simulink model "DOA_rearanged_2020a"  (R2020a)
settings: Solver=ode4  StartTime=0.0  StopTime=0.25  RelTol=1e-3
values from neighbouring files (symbols this model uses):
  f_range = [20e3 45e3]    [Init.m]
  FFT_LENGTH = 256    [Init.m]
  Sampling_rate = 256e3    (= 256000)    [Init.m]
undefined symbols (not defined in the file or in its folder): Coeff_han
libraries: dspsigops x25, dsphdlmathfun x4, dsphdlxfrm x4, simulink x1, hdlsllib x1
settings Model: Creator=tigro  LastModifiedBy=franc
settings OptimizationCC: BlockReduction=off  ConditionallyExecuteInputs=off  DefaultParameterBehavior=Inlined
settings DebuggingCC: AlgebraicLoopMsg=error  ParameterOverflowMsg=none  AllowAutomaticUnitConversions=off
settings HardwareCC: ProdBitPerPointer=32  ProdBitPerSizeT=32  ProdBitPerPtrDiffT=32  ProdLargestAtomicFloat=None  ProdIntDivRoundTo=Undefined  ProdEndianess=Unspecified  ProdWordSize=32  ProdHWDeviceType=ASIC/FPGA->ASIC/FPGA  TargetBitPerPointer=64  TargetBitPerSizeT=64  TargetBitPerPtrDiffT=64  TargetLongLongMode=on  TargetIntDivRoundTo=Zero  TargetEndianess=LittleEndian  TargetWordSize=64  TargetHWDeviceType=Custom Processor->MATLAB Host Computer  ProdEqTarget=off

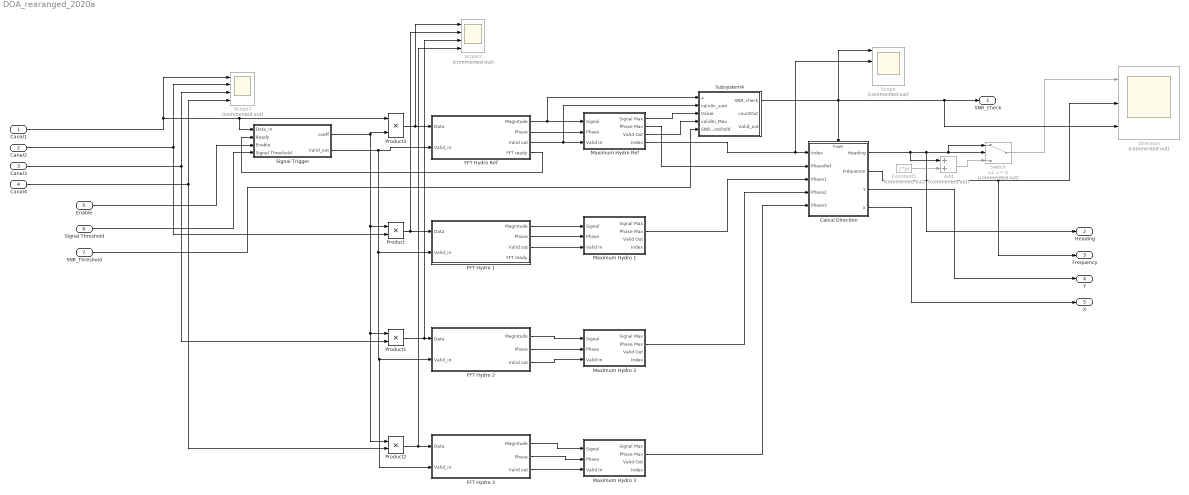
== system DOA_rearanged_2020a ==
  Canal1 : Inport  OutDataTypeStr=uint16
  Canal2 : Inport  Port=2  OutDataTypeStr=uint16
  Canal3 : Inport  Port=3  OutDataTypeStr=uint16
  Canal4 : Inport  Port=4  OutDataTypeStr=uint16
  Enable : Inport  Port=5  SampleTime=1/Sampling_rate
  Signal Threshold : Inport  Port=6
  SNR_Threshold : Inport  Port=7  OutDataTypeStr=uint16
  Add : Sum  Commented=on
  Calcul Direction : Subsystem
  Constant5 : Constant  Commented=on  Value=2*pi
  Direction : Scope  Commented=on  NumInputPorts=3
  FFT Hydro 1 : Subsystem
  FFT Hydro 2 : Subsystem
  FFT Hydro 3 : Subsystem
  FFT Hydro Ref : Subsystem
  Maximum Hydro 1 : Subsystem
  Maximum Hydro 2 : Subsystem
  Maximum Hydro 3 : Subsystem
  Maximum Hydro Ref : Subsystem
  Product{,1..3} (4 alike) : Product
  Scope : Scope  Commented=on  NumInputPorts=4
  Scope1 : Scope  Commented=on  NumInputPorts=4
  Scope2 : Scope  Commented=on  NumInputPorts=4
  Signal Trigger : Subsystem  TreatAsAtomicUnit=on
  Subsystem4 : Subsystem
  Switch : Switch  Commented=on
  SNR_Check : Outport
  Heading : Outport  Port=2
  Frequency : Outport  Port=3
  Y : Outport  Port=4
  X : Outport  Port=5
  wires:
  Maximum Hydro Ref/1(Signal Max) -> Subsystem4/3(" Value")
  Maximum Hydro Ref/4(Index) -> Scope/2, Calcul Direction/1(Index)
  Calcul Direction/1(Heading) -> Heading/1, Switch/2, Switch/1, Add/1
  Add/1 -> Switch/3
  Constant5/1 -> Add/2
  Product3/1 -> Scope2/1, FFT Hydro Ref/1(Data)
  Product/1 -> Scope2/2, FFT Hydro 1/1(Data)
  Product1/1 -> Scope2/3, FFT Hydro 2/1(Data)
  Product2/1 -> Scope2/4, FFT Hydro 3/1(Data)
  FFT Hydro Ref/2(Phase) -> Maximum Hydro Ref/2(Phase)
  Maximum Hydro Ref/2(Phase Max) -> Calcul Direction/2(PhaseRef)
  Maximum Hydro 1/2(Phase Max) -> Calcul Direction/3(Phase1)
  Maximum Hydro 2/2(Phase Max) -> Calcul Direction/4(Phase2)
  Maximum Hydro 3/2(Phase Max) -> Calcul Direction/5(Phase3)
  Signal Trigger/1(coeff) -> Product3/2, Product/1, Product1/1, Product2/1
  FFT Hydro 1/1(Magnitude) -> Maximum Hydro 1/1(Signal)
  FFT Hydro 1/2(Phase) -> Maximum Hydro 1/2(Phase)
  FFT Hydro 1/3(Valid out) -> Maximum Hydro 1/3(Valid In)
  FFT Hydro 2/2(Phase) -> Maximum Hydro 2/2(Phase)
  Maximum Hydro Ref/3(Valid Out) -> Subsystem4/4(validIn_Max)
  FFT Hydro Ref/4(FFT ready) -> Signal Trigger/2(Ready)
  FFT Hydro Ref/3(Valid out) -> Maximum Hydro Ref/3(Valid In), Subsystem4/2(validIn_sum)
  Calcul Direction/2(Fréquence) -> Frequency/1, Direction/2
  Calcul Direction/3(Y) -> Y/1
  Calcul Direction/4(X) -> X/1
  Switch/1 -> Direction/1
  FFT Hydro Ref/1(Magnitude) -> Subsystem4/1(a), Maximum Hydro Ref/1(Signal)
  Subsystem4/1(SNR_check) -> SNR_Check/1, Direction/3, Scope/1, Calcul Direction/Trigger
  Enable/1 -> Signal Trigger/3(Enable)
  Signal Threshold/1 -> Signal Trigger/4(Signal Threshold)
  SNR_Threshold/1 -> Subsystem4/5(SNR_Threshold)
  Signal Trigger/2(Valid_out) -> FFT Hydro 1/2(Valid_in), FFT Hydro 3/2(Valid_in), FFT Hydro 2/2(Valid_in), FFT Hydro Ref/2(Valid_in)
  Canal1/1 -> Scope1/1, Product3/1, Signal Trigger/1(Data_in)
  Canal2/1 -> Product/2, Scope1/2
  Canal3/1 -> Product1/2, Scope1/3
  Canal4/1 -> Product2/2, Scope1/4
  FFT Hydro 2/1(Magnitude) -> Maximum Hydro 2/1(Signal)
  FFT Hydro 2/3(Valid out) -> Maximum Hydro 2/3(Valid In)
  FFT Hydro 3/1(Magnitude) -> Maximum Hydro 3/1(Signal)
  FFT Hydro 3/2(Phase) -> Maximum Hydro 3/2(Phase)
  FFT Hydro 3/3(Valid out) -> Maximum Hydro 3/3(Valid In)

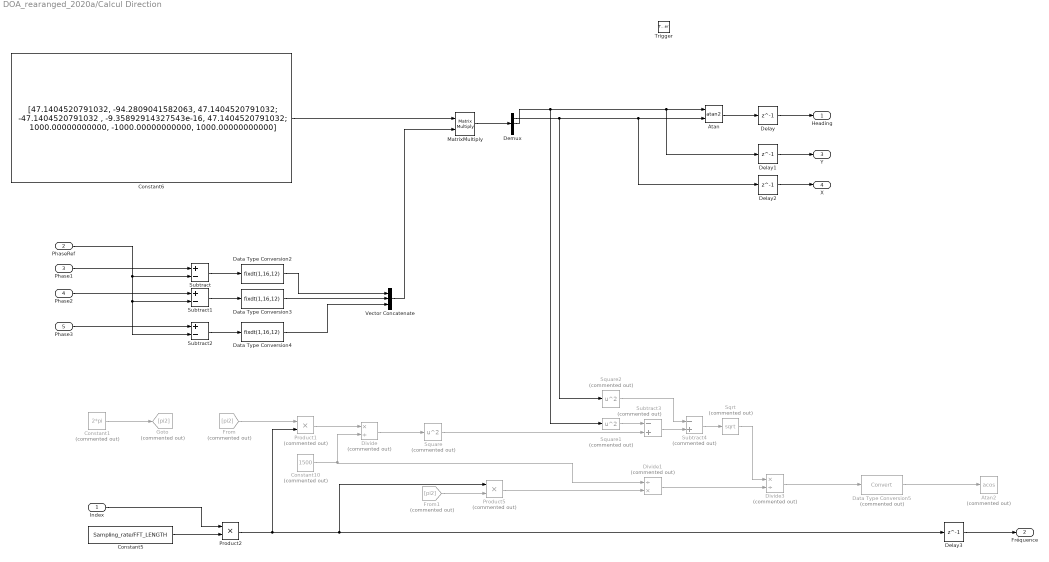
== system DOA_rearanged_2020a/Calcul Direction ==
  Index : Inport
  PhaseRef : Inport  Port=2
  Phase1 : Inport  Port=3
  Phase2 : Inport  Port=4
  Phase3 : Inport  Port=5
  Trigger : TriggerPort  VariantControl=Variant  PortDimensions=1
  Atan : Trigonometry  Operator=atan2  ApproximationMethod=CORDIC  OutputSignalType=real
  Atan2 : Trigonometry  Commented=on  Operator=acos  ApproximationMethod=CORDIC  OutputSignalType=real
  Constant1 : Constant  Commented=on  Value=2*pi  OutDataTypeStr=fixdt(0,7,3)  SampleTime=-1
  Constant10 : Constant  Commented=on  Value=1500  OutDataTypeStr=fixdt(0,11)  SampleTime=-1
  Constant5 : Constant  Value=Sampling_rate/FFT_LENGTH  OutDataTypeStr=fixdt(0,10)  SampleTime=-1
  Constant6 : Constant  Value=|  VectorParams1D=off  OutDataTypeStr=fixdt(1,15,7)  SampleTime=-1
      | [47.1404520791032,    -94.2809041582063,    47.1404520791032;
      | -47.1404520791032 ,   -9.35892914327543e-16,    47.1404520791032;
      | 1000.00000000000,   -1000.00000000000,    1000.00000000000]
  Data Type Conversion2 : DataTypeConversion  OutDataTypeStr=fixdt(1,16,12)
  Data Type Conversion3 : DataTypeConversion  OutDataTypeStr=fixdt(1,16,12)
  Data Type Conversion4 : DataTypeConversion  OutDataTypeStr=fixdt(1,16,12)
  Data Type Conversion5 : DataTypeConversion  Commented=on
  Delay{,1..3} (4 alike) : Delay  DelayLength=1
  Demux : Demux  Outputs=3
  Divide : Product  Commented=on  Inputs=*/
  Divide1 : Product  Commented=on  Inputs=/*
  Divide3 : Product  Commented=on  Inputs=*/
  From : From  Commented=on  GotoTag=pi2
  From1 : From  Commented=on  GotoTag=pi2
  Goto : Goto  Commented=on  GotoTag=pi2
  MatrixMultiply : Product  Multiplication=Matrix(*)
  Product1 : Product  Commented=on
  Product2 : Product
  Product5 : Product  Commented=on
  Sqrt : Sqrt  Commented=on  SaturateOnIntegerOverflow=on
  Square : Math  Commented=on  Operator=square  SignedPower=on  RndMeth=Zero  SaturateOnIntegerOverflow=on
  Square1 : Math  Commented=on  Operator=square  SignedPower=on  RndMeth=Zero  SaturateOnIntegerOverflow=on
  Square2 : Math  Commented=on  Operator=square  SignedPower=on  RndMeth=Zero  SaturateOnIntegerOverflow=on
  Subtract : Sum  Inputs=+-
  Subtract1 : Sum  Inputs=+-
  Subtract2 : Sum  Inputs=+-
  Subtract3 : Sum  Commented=on  Inputs=-+
  Subtract4 : Sum  Commented=on  Inputs=-+
  Vector Concatenate : Concatenate  NumInputs=3  Mode=Multidimensional array
  Heading : Outport  InitialOutput=0
  Fréquence : Outport  Port=2  InitialOutput=0
  Y : Outport  Port=3  InitialOutput=0
  X : Outport  Port=4  InitialOutput=0
  wires:
  Vector Concatenate/1 -> MatrixMultiply/2
  MatrixMultiply/1 -> Demux/1
  PhaseRef/1 -> Subtract/2, Subtract1/2, Subtract2/2
  Phase1/1 -> Subtract/1
  Phase2/1 -> Subtract1/1
  Phase3/1 -> Subtract2/1
  Subtract/1 -> Data Type Conversion2/1
  Subtract1/1 -> Data Type Conversion3/1
  Subtract2/1 -> Data Type Conversion4/1
  Constant6/1 -> MatrixMultiply/1
  Sqrt/1 -> Divide3/1
  Divide/1 -> Square/1
  From/1 -> Product1/1
  Demux/2 -> Square1/1, Delay1/1, Atan/1
  Constant1/1 -> Goto/1
  Divide1/1 -> Divide3/2
  Product5/1 -> Divide1/2
  From1/1 -> Product5/2
  Constant10/1 -> Divide/2, Divide1/1
  Subtract3/1 -> Subtract4/2
  Product1/1 -> Divide/1
  Square1/1 -> Subtract3/1
  Square/1 -> Subtract3/2
  Subtract4/1 -> Sqrt/1
  Constant5/1 -> Product2/2
  Index/1 -> Product2/1
  Square2/1 -> Subtract4/1
  Demux/1 -> Square2/1, Delay2/1, Atan/2
  Divide3/1 -> Data Type Conversion5/1
  Product2/1 -> Delay3/1, Product5/1, Product1/2
  Data Type Conversion2/1 -> Vector Concatenate/1
  Data Type Conversion3/1 -> Vector Concatenate/2
  Data Type Conversion4/1 -> Vector Concatenate/3
  Data Type Conversion5/1 -> Atan2/1
  Atan/1 -> Delay/1
  Delay/1 -> Heading/1
  Delay2/1 -> X/1
  Delay1/1 -> Y/1
  Delay3/1 -> Fréquence/1

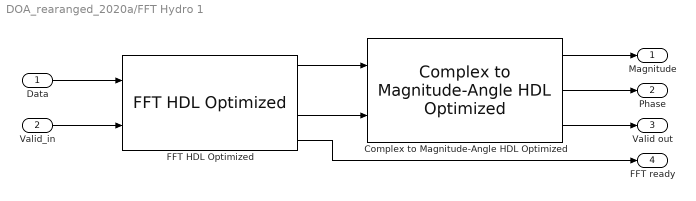
== system DOA_rearanged_2020a/FFT Hydro 1 ==
  Data : Inport
  Valid_in : Inport  Port=2
  Complex to Magnitude-Angle HDL Optimized : dsphdlmathfun/Complex to Magnitude-Angle HDL Optimized  NumIterationsSource=Property  NumIterations=CORDIC_Estimation  OutputFormat=Magnitude and angle  AngleFormat=Radians  ScaleOutput=on  SimulateUsing=Code generation
      settings: SourceProductBaseCode=DS
  FFT HDL Optimized : dsphdlxfrm/FFT HDL Optimized  FFTLength=FFT_LENGTH  Architecture=Burst Radix 2  ComplexMultiplication=Use 3 multipliers and 5 adders  BitReversedOutput=off  BitReversedInput=off  Normalize=on  SimulateUsing=Code generation  RoundingMethod=Floor  ResetInputPort=off  StartOutputPort=off  EndOutputPort=on
      settings: SourceProductBaseCode=DS
  Magnitude : Outport
  Phase : Outport  Port=2
  Valid out : Outport  Port=3
  FFT ready : Outport  Port=4
  wires:
  Valid_in/1 -> FFT HDL Optimized/2
  FFT HDL Optimized/1 -> Complex to Magnitude-Angle HDL Optimized/1
  Complex to Magnitude-Angle HDL Optimized/1 -> Magnitude/1
  Complex to Magnitude-Angle HDL Optimized/2 -> Phase/1
  Data/1 -> FFT HDL Optimized/1
  FFT HDL Optimized/3 -> Complex to Magnitude-Angle HDL Optimized/2
  Complex to Magnitude-Angle HDL Optimized/3 -> Valid out/1
  FFT HDL Optimized/4 -> FFT ready/1

== system DOA_rearanged_2020a/FFT Hydro 2 ==
  Data : Inport
  Valid_in : Inport  Port=2
  Complex to Magnitude-Angle HDL Optimized : dsphdlmathfun/Complex to Magnitude-Angle HDL Optimized  NumIterationsSource=Property  NumIterations=CORDIC_Estimation  OutputFormat=Magnitude and angle  AngleFormat=Radians  ScaleOutput=on  SimulateUsing=Code generation
      settings: SourceProductBaseCode=DS
  FFT HDL Optimized : dsphdlxfrm/FFT HDL Optimized  FFTLength=FFT_LENGTH  Architecture=Burst Radix 2  ComplexMultiplication=Use 3 multipliers and 5 adders  BitReversedOutput=off  BitReversedInput=off  Normalize=on  SimulateUsing=Code generation  RoundingMethod=Floor  ResetInputPort=off  StartOutputPort=off  EndOutputPort=off
      settings: SourceProductBaseCode=DS
  Magnitude : Outport
  Phase : Outport  Port=2
  Valid out : Outport  Port=3
  wires:
  Valid_in/1 -> FFT HDL Optimized/2
  FFT HDL Optimized/1 -> Complex to Magnitude-Angle HDL Optimized/1
  FFT HDL Optimized/2 -> Complex to Magnitude-Angle HDL Optimized/2
  Complex to Magnitude-Angle HDL Optimized/1 -> Magnitude/1
  Complex to Magnitude-Angle HDL Optimized/3 -> Valid out/1
  Complex to Magnitude-Angle HDL Optimized/2 -> Phase/1
  Data/1 -> FFT HDL Optimized/1

== system DOA_rearanged_2020a/FFT Hydro 3 ==
  Data : Inport
  Valid_in : Inport  Port=2
  Complex to Magnitude-Angle HDL Optimized : dsphdlmathfun/Complex to Magnitude-Angle HDL Optimized  NumIterationsSource=Property  NumIterations=CORDIC_Estimation  OutputFormat=Magnitude and angle  AngleFormat=Radians  ScaleOutput=on  SimulateUsing=Code generation
      settings: SourceProductBaseCode=DS
  FFT HDL Optimized : dsphdlxfrm/FFT HDL Optimized  FFTLength=FFT_LENGTH  Architecture=Burst Radix 2  ComplexMultiplication=Use 3 multipliers and 5 adders  BitReversedOutput=off  BitReversedInput=off  Normalize=on  SimulateUsing=Code generation  RoundingMethod=Floor  ResetInputPort=off  StartOutputPort=off  EndOutputPort=off
      settings: SourceProductBaseCode=DS
  Magnitude : Outport
  Phase : Outport  Port=2
  Valid out : Outport  Port=3
  wires:
  Valid_in/1 -> FFT HDL Optimized/2
  FFT HDL Optimized/1 -> Complex to Magnitude-Angle HDL Optimized/1
  FFT HDL Optimized/2 -> Complex to Magnitude-Angle HDL Optimized/2
  Complex to Magnitude-Angle HDL Optimized/1 -> Magnitude/1
  Complex to Magnitude-Angle HDL Optimized/3 -> Valid out/1
  Complex to Magnitude-Angle HDL Optimized/2 -> Phase/1
  Data/1 -> FFT HDL Optimized/1

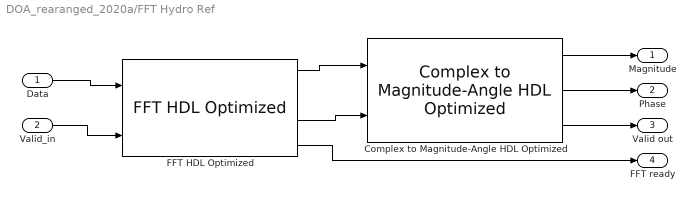
== system DOA_rearanged_2020a/FFT Hydro Ref ==
  Data : Inport
  Valid_in : Inport  Port=2
  Complex to Magnitude-Angle HDL Optimized : dsphdlmathfun/Complex to Magnitude-Angle HDL Optimized  NumIterationsSource=Property  NumIterations=CORDIC_Estimation  OutputFormat=Magnitude and angle  AngleFormat=Radians  ScaleOutput=on  SimulateUsing=Code generation
      settings: SourceProductBaseCode=DS
  FFT HDL Optimized : dsphdlxfrm/FFT HDL Optimized  FFTLength=FFT_LENGTH  Architecture=Burst Radix 2  ComplexMultiplication=Use 3 multipliers and 5 adders  BitReversedOutput=off  BitReversedInput=off  Normalize=on  SimulateUsing=Code generation  RoundingMethod=Floor  ResetInputPort=off  StartOutputPort=off  EndOutputPort=on
      settings: SourceProductBaseCode=DS
  Magnitude : Outport
  Phase : Outport  Port=2
  Valid out : Outport  Port=3
  FFT ready : Outport  Port=4
  wires:
  Valid_in/1 -> FFT HDL Optimized/2
  FFT HDL Optimized/1 -> Complex to Magnitude-Angle HDL Optimized/1
  Complex to Magnitude-Angle HDL Optimized/1 -> Magnitude/1
  Complex to Magnitude-Angle HDL Optimized/2 -> Phase/1
  Data/1 -> FFT HDL Optimized/1
  FFT HDL Optimized/3 -> Complex to Magnitude-Angle HDL Optimized/2
  Complex to Magnitude-Angle HDL Optimized/3 -> Valid out/1
  FFT HDL Optimized/4 -> FFT ready/1

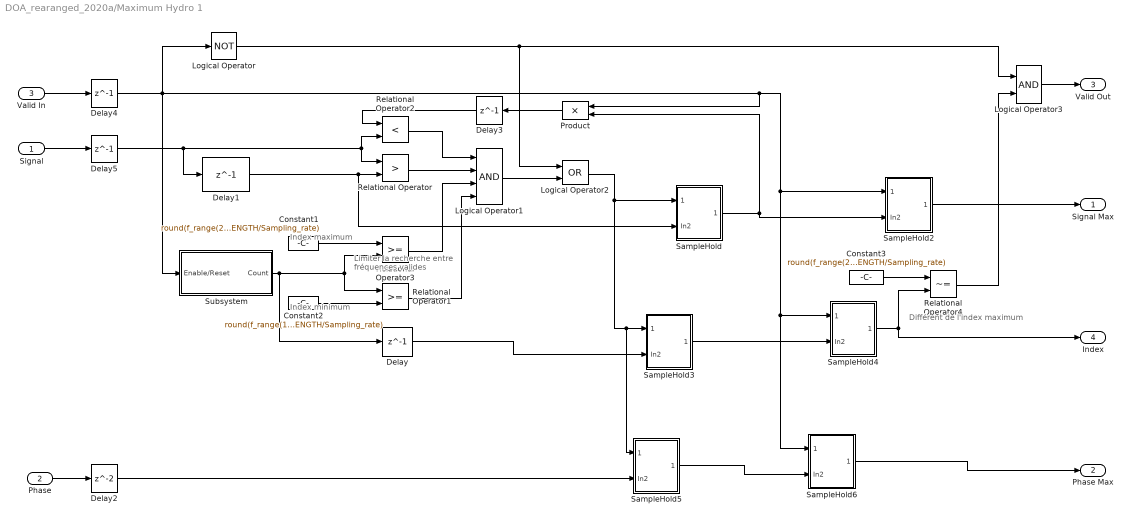
== system DOA_rearanged_2020a/Maximum Hydro 1 ==
  note: Index minimum
  note: Index maximum
  note: Limiter la recherche
      | entre fréquences valides
  note: Différent de l'index
      | maximum
  Signal : Inport
  Phase : Inport  Port=2
  Valid In : Inport  Port=3
  Constant1 : Constant  Value=round(f_range(2)*FFT_LENGTH/Sampling_rate)  OutDataTypeStr=fixdt(0,6)  SampleTime=-1
  Constant2 : Constant  Value=round(f_range(1)*FFT_LENGTH/Sampling_rate)  OutDataTypeStr=fixdt(0,6)  SampleTime=-1
  Constant3 : Constant  Value=round(f_range(2)*FFT_LENGTH/Sampling_rate)  OutDataTypeStr=fixdt(0,6)  SampleTime=-1
  Delay : Delay  DelayLength=1  InitialCondition=0
  Delay{1,3..5} (4 alike) : Delay  DelayLength=1  InitialCondition=0  UseCircularBuffer=on
  Delay2 : Delay  InitialCondition=0  UseCircularBuffer=on
  Logical Operator : Logic  Operator=NOT  IconShape=distinctive  AllPortsSameDT=off  OutDataTypeStr=boolean
  Logical Operator1 : Logic  Inputs=4  AllPortsSameDT=off  OutDataTypeStr=boolean
  Logical Operator2 : Logic  Operator=OR  AllPortsSameDT=off  OutDataTypeStr=boolean
  Logical Operator3 : Logic  AllPortsSameDT=off  OutDataTypeStr=boolean
  Product : Product
  Relational Operator : RelationalOperator  Operator=>  OutDataTypeStr=boolean  RndMeth=Nearest
  Relational Operator1 : RelationalOperator  OutDataTypeStr=boolean  RndMeth=Nearest
  Relational Operator2 : RelationalOperator  Operator=<  OutDataTypeStr=boolean  RndMeth=Nearest
  Relational Operator3 : RelationalOperator  OutDataTypeStr=boolean  RndMeth=Nearest
  Relational Operator4 : RelationalOperator  Operator=~=  OutDataTypeStr=boolean  RndMeth=Nearest
  SampleHold : Subsystem  TreatAsAtomicUnit=on
  SampleHold2 : Subsystem  TreatAsAtomicUnit=on
  SampleHold3 : Subsystem  TreatAsAtomicUnit=on
  SampleHold4 : Subsystem  TreatAsAtomicUnit=on
  SampleHold5 : Subsystem  TreatAsAtomicUnit=on
  SampleHold6 : Subsystem  TreatAsAtomicUnit=on
  Subsystem : Subsystem
  Signal Max : Outport  VectorParamsAs1DForOutWhenUnconnected=off
  Phase Max : Outport  Port=2  VectorParamsAs1DForOutWhenUnconnected=off
  Valid Out : Outport  Port=3  VectorParamsAs1DForOutWhenUnconnected=off
  Index : Outport  Port=4  VectorParamsAs1DForOutWhenUnconnected=off
  wires:
  SampleHold/1(" ") -> SampleHold2/2(In2), Product/2
  Signal/1 -> Delay5/1
  SampleHold3/1(" ") -> SampleHold4/2(In2)
  Valid In/1 -> Delay4/1
  Delay1/1 -> SampleHold/2(In2), Relational Operator/2
  SampleHold2/1(" ") -> Signal Max/1
  Constant2/1 -> Relational Operator1/2
  SampleHold5/1(" ") -> SampleHold6/2(In2)
  Phase/1 -> Delay2/1
  SampleHold6/1(" ") -> Phase Max/1
  Subsystem/1(Count) -> Delay/1, Relational Operator1/1, Relational Operator3/2
  Relational Operator2/1 -> Logical Operator1/1
  Relational Operator/1 -> Logical Operator1/2
  Delay3/1 -> Relational Operator2/1
  Product/1 -> Delay3/1
  Delay4/1 -> Logical Operator/1, SampleHold6/1(Trigger), SampleHold4/1(Trigger), SampleHold2/1(Trigger), Product/1, Subsystem/1(Enable/Reset)
  Delay5/1 -> Relational Operator2/2, Relational Operator/1, Delay1/1
  Delay2/1 -> SampleHold5/2(In2)
  Constant1/1 -> Relational Operator3/1
  Relational Operator1/1 -> Logical Operator1/4
  Logical Operator/1 -> Logical Operator2/1, Logical Operator3/1
  Logical Operator3/1 -> Valid Out/1
  Relational Operator3/1 -> Logical Operator1/3
  Relational Operator4/1 -> Logical Operator3/2
  SampleHold4/1(" ") -> Index/1, Relational Operator4/2
  Constant3/1 -> Relational Operator4/1
  Logical Operator1/1 -> Logical Operator2/2
  Logical Operator2/1 -> SampleHold5/1(Trigger), SampleHold3/1(Trigger), SampleHold/1(Trigger)
  Delay/1 -> SampleHold3/2(In2)

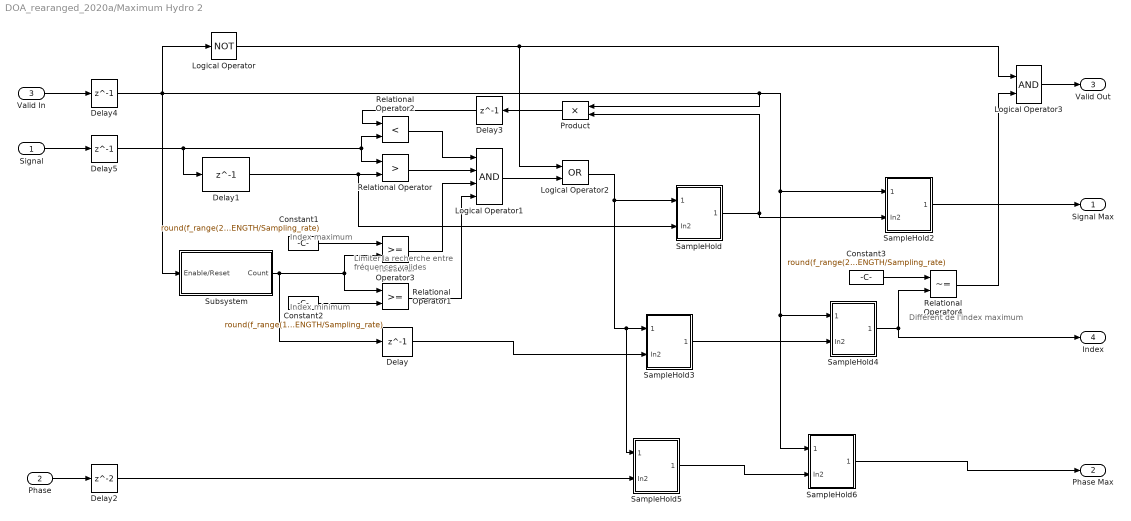
== system DOA_rearanged_2020a/Maximum Hydro 2 ==
  note: Index minimum
  note: Index maximum
  note: Limiter la recherche
      | entre fréquences valides
  note: Différent de l'index
      | maximum
  Signal : Inport
  Phase : Inport  Port=2
  Valid In : Inport  Port=3
  Constant1 : Constant  Value=round(f_range(2)*FFT_LENGTH/Sampling_rate)  OutDataTypeStr=fixdt(0,6)  SampleTime=-1
  Constant2 : Constant  Value=round(f_range(1)*FFT_LENGTH/Sampling_rate)  OutDataTypeStr=fixdt(0,6)  SampleTime=-1
  Constant3 : Constant  Value=round(f_range(2)*FFT_LENGTH/Sampling_rate)  OutDataTypeStr=fixdt(0,6)  SampleTime=-1
  Delay : Delay  DelayLength=1  InitialCondition=0
  Delay{1,3..5} (4 alike) : Delay  DelayLength=1  InitialCondition=0  UseCircularBuffer=on
  Delay2 : Delay  InitialCondition=0  UseCircularBuffer=on
  Logical Operator : Logic  Operator=NOT  IconShape=distinctive  AllPortsSameDT=off  OutDataTypeStr=boolean
  Logical Operator1 : Logic  Inputs=4  AllPortsSameDT=off  OutDataTypeStr=boolean
  Logical Operator2 : Logic  Operator=OR  AllPortsSameDT=off  OutDataTypeStr=boolean
  Logical Operator3 : Logic  AllPortsSameDT=off  OutDataTypeStr=boolean
  Product : Product
  Relational Operator : RelationalOperator  Operator=>  OutDataTypeStr=boolean  RndMeth=Nearest
  Relational Operator1 : RelationalOperator  OutDataTypeStr=boolean  RndMeth=Nearest
  Relational Operator2 : RelationalOperator  Operator=<  OutDataTypeStr=boolean  RndMeth=Nearest
  Relational Operator3 : RelationalOperator  OutDataTypeStr=boolean  RndMeth=Nearest
  Relational Operator4 : RelationalOperator  Operator=~=  OutDataTypeStr=boolean  RndMeth=Nearest
  SampleHold : Subsystem  TreatAsAtomicUnit=on
  SampleHold2 : Subsystem  TreatAsAtomicUnit=on
  SampleHold3 : Subsystem  TreatAsAtomicUnit=on
  SampleHold4 : Subsystem  TreatAsAtomicUnit=on
  SampleHold5 : Subsystem  TreatAsAtomicUnit=on
  SampleHold6 : Subsystem  TreatAsAtomicUnit=on
  Subsystem : Subsystem
  Signal Max : Outport  VectorParamsAs1DForOutWhenUnconnected=off
  Phase Max : Outport  Port=2  VectorParamsAs1DForOutWhenUnconnected=off
  Valid Out : Outport  Port=3  VectorParamsAs1DForOutWhenUnconnected=off
  Index : Outport  Port=4  VectorParamsAs1DForOutWhenUnconnected=off
  wires:
  SampleHold/1(" ") -> SampleHold2/2(In2), Product/2
  Signal/1 -> Delay5/1
  SampleHold3/1(" ") -> SampleHold4/2(In2)
  Valid In/1 -> Delay4/1
  Delay1/1 -> SampleHold/2(In2), Relational Operator/2
  SampleHold2/1(" ") -> Signal Max/1
  Constant2/1 -> Relational Operator1/2
  SampleHold5/1(" ") -> SampleHold6/2(In2)
  Phase/1 -> Delay2/1
  SampleHold6/1(" ") -> Phase Max/1
  Subsystem/1(Count) -> Delay/1, Relational Operator1/1, Relational Operator3/2
  Relational Operator2/1 -> Logical Operator1/1
  Relational Operator/1 -> Logical Operator1/2
  Delay3/1 -> Relational Operator2/1
  Product/1 -> Delay3/1
  Delay4/1 -> Logical Operator/1, SampleHold6/1(Trigger), SampleHold4/1(Trigger), SampleHold2/1(Trigger), Product/1, Subsystem/1(Enable/Reset)
  Delay5/1 -> Relational Operator2/2, Relational Operator/1, Delay1/1
  Delay2/1 -> SampleHold5/2(In2)
  Constant1/1 -> Relational Operator3/1
  Relational Operator1/1 -> Logical Operator1/4
  Logical Operator/1 -> Logical Operator2/1, Logical Operator3/1
  Logical Operator3/1 -> Valid Out/1
  Relational Operator3/1 -> Logical Operator1/3
  Relational Operator4/1 -> Logical Operator3/2
  SampleHold4/1(" ") -> Index/1, Relational Operator4/2
  Constant3/1 -> Relational Operator4/1
  Logical Operator1/1 -> Logical Operator2/2
  Logical Operator2/1 -> SampleHold5/1(Trigger), SampleHold3/1(Trigger), SampleHold/1(Trigger)
  Delay/1 -> SampleHold3/2(In2)

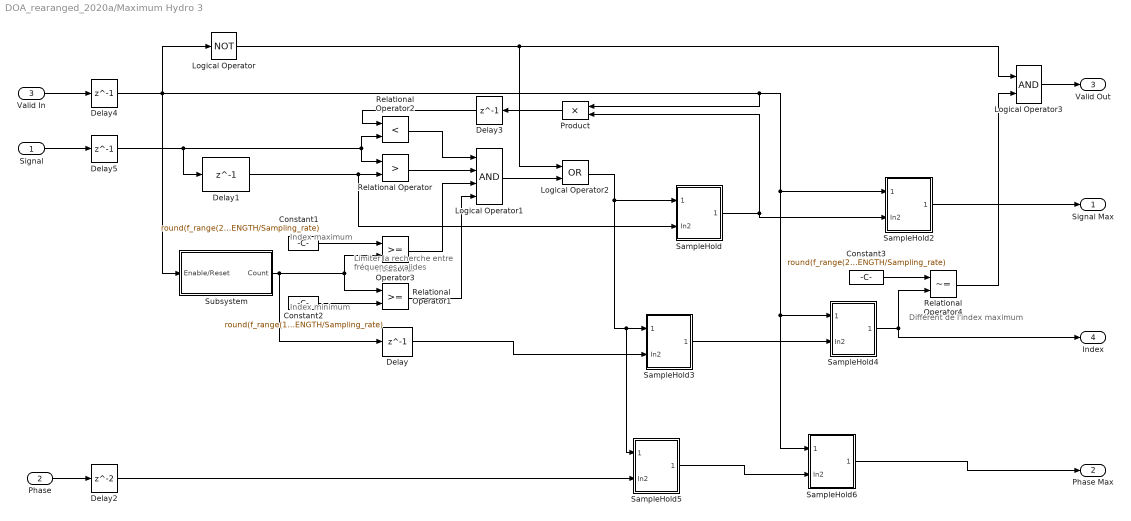
== system DOA_rearanged_2020a/Maximum Hydro 3 ==
  note: Index minimum
  note: Index maximum
  note: Limiter la recherche
      | entre fréquences valides
  note: Différent de l'index
      | maximum
  Signal : Inport
  Phase : Inport  Port=2
  Valid In : Inport  Port=3
  Constant1 : Constant  Value=round(f_range(2)*FFT_LENGTH/Sampling_rate)  OutDataTypeStr=fixdt(0,6)  SampleTime=-1
  Constant2 : Constant  Value=round(f_range(1)*FFT_LENGTH/Sampling_rate)  OutDataTypeStr=fixdt(0,6)  SampleTime=-1
  Constant3 : Constant  Value=round(f_range(2)*FFT_LENGTH/Sampling_rate)  OutDataTypeStr=fixdt(0,6)  SampleTime=-1
  Delay : Delay  DelayLength=1  InitialCondition=0
  Delay{1,3..5} (4 alike) : Delay  DelayLength=1  InitialCondition=0  UseCircularBuffer=on
  Delay2 : Delay  InitialCondition=0  UseCircularBuffer=on
  Logical Operator : Logic  Operator=NOT  IconShape=distinctive  AllPortsSameDT=off  OutDataTypeStr=boolean
  Logical Operator1 : Logic  Inputs=4  AllPortsSameDT=off  OutDataTypeStr=boolean
  Logical Operator2 : Logic  Operator=OR  AllPortsSameDT=off  OutDataTypeStr=boolean
  Logical Operator3 : Logic  AllPortsSameDT=off  OutDataTypeStr=boolean
  Product : Product
  Relational Operator : RelationalOperator  Operator=>  OutDataTypeStr=boolean  RndMeth=Nearest
  Relational Operator1 : RelationalOperator  OutDataTypeStr=boolean  RndMeth=Nearest
  Relational Operator2 : RelationalOperator  Operator=<  OutDataTypeStr=boolean  RndMeth=Nearest
  Relational Operator3 : RelationalOperator  OutDataTypeStr=boolean  RndMeth=Nearest
  Relational Operator4 : RelationalOperator  Operator=~=  OutDataTypeStr=boolean  RndMeth=Nearest
  SampleHold : Subsystem  TreatAsAtomicUnit=on
  SampleHold2 : Subsystem  TreatAsAtomicUnit=on
  SampleHold3 : Subsystem  TreatAsAtomicUnit=on
  SampleHold4 : Subsystem  TreatAsAtomicUnit=on
  SampleHold5 : Subsystem  TreatAsAtomicUnit=on
  SampleHold6 : Subsystem  TreatAsAtomicUnit=on
  Subsystem : Subsystem
  Signal Max : Outport  VectorParamsAs1DForOutWhenUnconnected=off
  Phase Max : Outport  Port=2  VectorParamsAs1DForOutWhenUnconnected=off
  Valid Out : Outport  Port=3  VectorParamsAs1DForOutWhenUnconnected=off
  Index : Outport  Port=4  VectorParamsAs1DForOutWhenUnconnected=off
  wires:
  SampleHold/1(" ") -> SampleHold2/2(In2), Product/2
  Signal/1 -> Delay5/1
  SampleHold3/1(" ") -> SampleHold4/2(In2)
  Valid In/1 -> Delay4/1
  Delay1/1 -> SampleHold/2(In2), Relational Operator/2
  SampleHold2/1(" ") -> Signal Max/1
  Constant2/1 -> Relational Operator1/2
  SampleHold5/1(" ") -> SampleHold6/2(In2)
  Phase/1 -> Delay2/1
  SampleHold6/1(" ") -> Phase Max/1
  Subsystem/1(Count) -> Delay/1, Relational Operator1/1, Relational Operator3/2
  Relational Operator2/1 -> Logical Operator1/1
  Relational Operator/1 -> Logical Operator1/2
  Delay3/1 -> Relational Operator2/1
  Product/1 -> Delay3/1
  Delay4/1 -> Logical Operator/1, SampleHold6/1(Trigger), SampleHold4/1(Trigger), SampleHold2/1(Trigger), Product/1, Subsystem/1(Enable/Reset)
  Delay5/1 -> Relational Operator2/2, Relational Operator/1, Delay1/1
  Delay2/1 -> SampleHold5/2(In2)
  Constant1/1 -> Relational Operator3/1
  Relational Operator1/1 -> Logical Operator1/4
  Logical Operator/1 -> Logical Operator2/1, Logical Operator3/1
  Logical Operator3/1 -> Valid Out/1
  Relational Operator3/1 -> Logical Operator1/3
  Relational Operator4/1 -> Logical Operator3/2
  SampleHold4/1(" ") -> Index/1, Relational Operator4/2
  Constant3/1 -> Relational Operator4/1
  Logical Operator1/1 -> Logical Operator2/2
  Logical Operator2/1 -> SampleHold5/1(Trigger), SampleHold3/1(Trigger), SampleHold/1(Trigger)
  Delay/1 -> SampleHold3/2(In2)

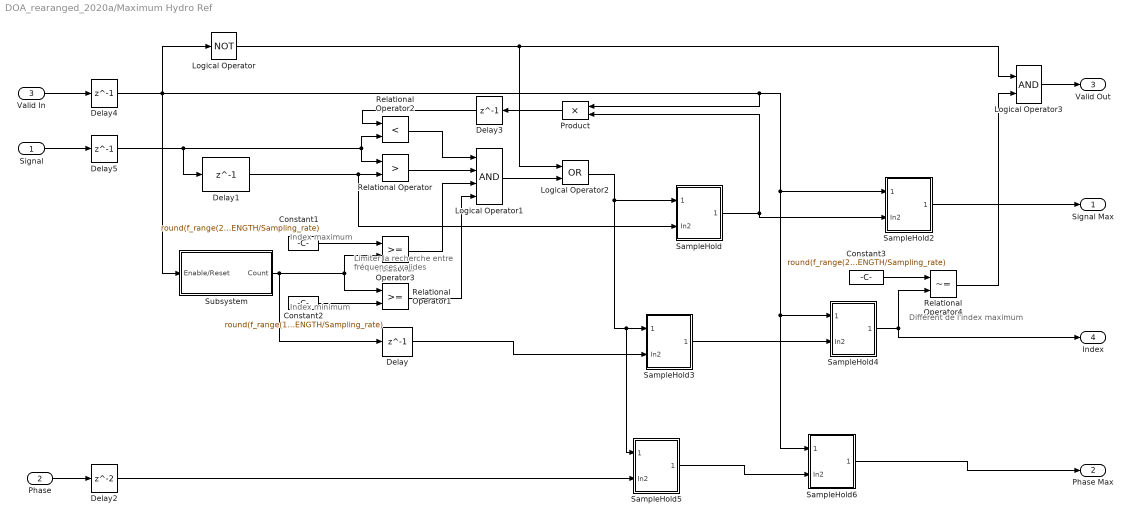
== system DOA_rearanged_2020a/Maximum Hydro Ref ==
  note: Index minimum
  note: Index maximum
  note: Limiter la recherche
      | entre fréquences valides
  note: Différent de l'index
      | maximum
  Signal : Inport
  Phase : Inport  Port=2
  Valid In : Inport  Port=3
  Constant1 : Constant  Value=round(f_range(2)*FFT_LENGTH/Sampling_rate)  OutDataTypeStr=fixdt(0,6)  SampleTime=-1
  Constant2 : Constant  Value=round(f_range(1)*FFT_LENGTH/Sampling_rate)  OutDataTypeStr=fixdt(0,6)  SampleTime=-1
  Constant3 : Constant  Value=round(f_range(2)*FFT_LENGTH/Sampling_rate)  OutDataTypeStr=fixdt(0,6)  SampleTime=-1
  Delay : Delay  DelayLength=1  InitialCondition=0
  Delay{1,3..5} (4 alike) : Delay  DelayLength=1  InitialCondition=0  UseCircularBuffer=on
  Delay2 : Delay  InitialCondition=0  UseCircularBuffer=on
  Logical Operator : Logic  Operator=NOT  IconShape=distinctive  AllPortsSameDT=off  OutDataTypeStr=boolean
  Logical Operator1 : Logic  Inputs=4  AllPortsSameDT=off  OutDataTypeStr=boolean
  Logical Operator2 : Logic  Operator=OR  AllPortsSameDT=off  OutDataTypeStr=boolean
  Logical Operator3 : Logic  AllPortsSameDT=off  OutDataTypeStr=boolean
  Product : Product
  Relational Operator : RelationalOperator  Operator=>  OutDataTypeStr=boolean  RndMeth=Nearest
  Relational Operator1 : RelationalOperator  OutDataTypeStr=boolean  RndMeth=Nearest
  Relational Operator2 : RelationalOperator  Operator=<  OutDataTypeStr=boolean  RndMeth=Nearest
  Relational Operator3 : RelationalOperator  OutDataTypeStr=boolean  RndMeth=Nearest
  Relational Operator4 : RelationalOperator  Operator=~=  OutDataTypeStr=boolean  RndMeth=Nearest
  SampleHold : Subsystem  TreatAsAtomicUnit=on
  SampleHold2 : Subsystem  TreatAsAtomicUnit=on
  SampleHold3 : Subsystem  TreatAsAtomicUnit=on
  SampleHold4 : Subsystem  TreatAsAtomicUnit=on
  SampleHold5 : Subsystem  TreatAsAtomicUnit=on
  SampleHold6 : Subsystem  TreatAsAtomicUnit=on
  Subsystem : Subsystem
  Signal Max : Outport  VectorParamsAs1DForOutWhenUnconnected=off
  Phase Max : Outport  Port=2  VectorParamsAs1DForOutWhenUnconnected=off
  Valid Out : Outport  Port=3  VectorParamsAs1DForOutWhenUnconnected=off
  Index : Outport  Port=4  VectorParamsAs1DForOutWhenUnconnected=off
  wires:
  SampleHold/1(" ") -> SampleHold2/2(In2), Product/2
  Signal/1 -> Delay5/1
  SampleHold3/1(" ") -> SampleHold4/2(In2)
  Valid In/1 -> Delay4/1
  Delay1/1 -> SampleHold/2(In2), Relational Operator/2
  SampleHold2/1(" ") -> Signal Max/1
  Constant2/1 -> Relational Operator1/2
  SampleHold5/1(" ") -> SampleHold6/2(In2)
  Phase/1 -> Delay2/1
  SampleHold6/1(" ") -> Phase Max/1
  Subsystem/1(Count) -> Delay/1, Relational Operator1/1, Relational Operator3/2
  Relational Operator2/1 -> Logical Operator1/1
  Relational Operator/1 -> Logical Operator1/2
  Delay3/1 -> Relational Operator2/1
  Product/1 -> Delay3/1
  Delay4/1 -> Logical Operator/1, SampleHold6/1(Trigger), SampleHold4/1(Trigger), SampleHold2/1(Trigger), Product/1, Subsystem/1(Enable/Reset)
  Delay5/1 -> Relational Operator2/2, Relational Operator/1, Delay1/1
  Delay2/1 -> SampleHold5/2(In2)
  Constant1/1 -> Relational Operator3/1
  Relational Operator1/1 -> Logical Operator1/4
  Logical Operator/1 -> Logical Operator2/1, Logical Operator3/1
  Logical Operator3/1 -> Valid Out/1
  Relational Operator3/1 -> Logical Operator1/3
  Relational Operator4/1 -> Logical Operator3/2
  SampleHold4/1(" ") -> Index/1, Relational Operator4/2
  Constant3/1 -> Relational Operator4/1
  Logical Operator1/1 -> Logical Operator2/2
  Logical Operator2/1 -> SampleHold5/1(Trigger), SampleHold3/1(Trigger), SampleHold/1(Trigger)
  Delay/1 -> SampleHold3/2(In2)

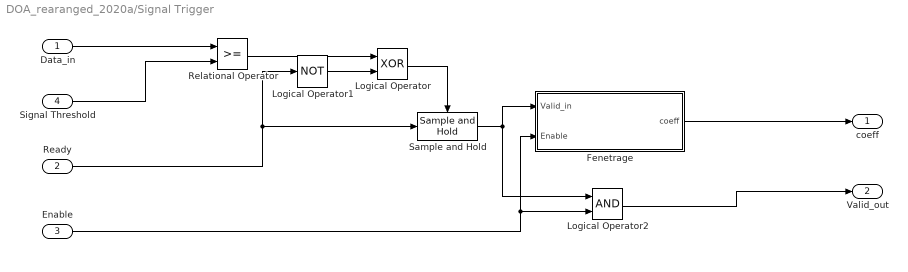
== system DOA_rearanged_2020a/Signal Trigger ==
  Data_in : Inport
  Ready : Inport  Port=2  OutDataTypeStr=boolean
  Enable : Inport  Port=3  OutDataTypeStr=boolean
  Signal Threshold : Inport  Port=4
  Fenetrage : Subsystem
  Logical Operator : Logic  Operator=XOR  AllPortsSameDT=off  OutDataTypeStr=boolean
  Logical Operator1 : Logic  Operator=NOT  IconShape=distinctive  AllPortsSameDT=off  OutDataTypeStr=boolean
  Logical Operator2 : Logic  AllPortsSameDT=off  OutDataTypeStr=boolean
  Relational Operator : RelationalOperator  OutDataTypeStr=boolean  RndMeth=Nearest
  Sample and Hold : dspsigops/Sample and Hold  trig=Rising edge  initCond=0  latchinput=off
  coeff : Outport
  Valid_out : Outport  Port=2
  wires:
  Data_in/1 -> Relational Operator/1
  Fenetrage/1(coeff) -> coeff/1
  Relational Operator/1 -> Logical Operator/1
  Ready/1 -> Logical Operator1/1, Sample and Hold/1
  Logical Operator/1 -> Sample and Hold/Trigger
  Sample and Hold/1 -> Logical Operator2/1, Fenetrage/1(Valid_in)
  Logical Operator1/1 -> Logical Operator/2
  Enable/1 -> Logical Operator2/2, Fenetrage/2(Enable)
  Logical Operator2/1 -> Valid_out/1
  Signal Threshold/1 -> Relational Operator/2

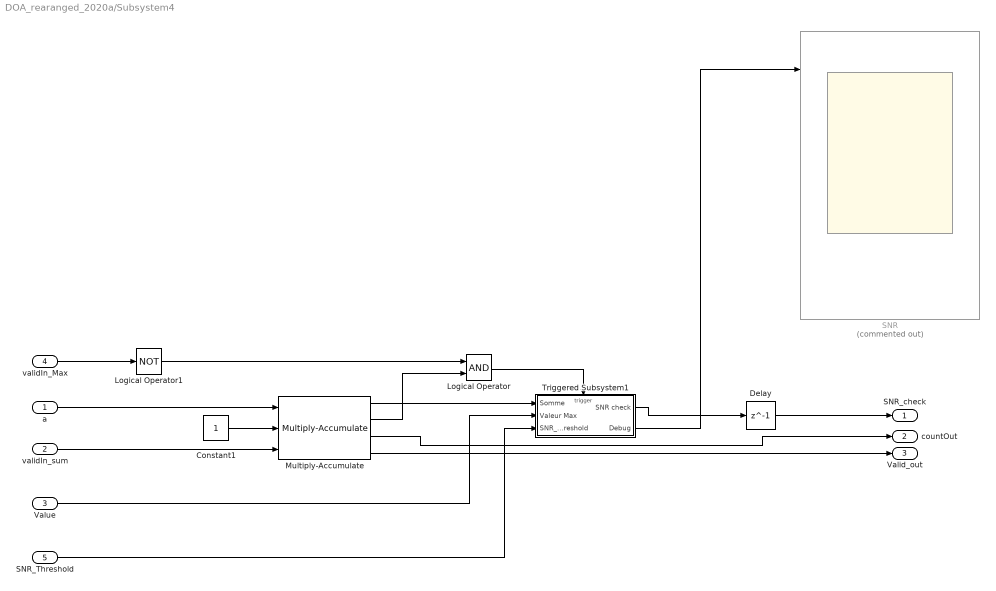
== system DOA_rearanged_2020a/Subsystem4 ==
  a : Inport
  validIn_sum : Inport  Port=2
  " Value" : Inport  Port=3
  validIn_Max : Inport  Port=4
  SNR_Threshold : Inport  Port=5
  Constant1 : Constant  OutDataTypeStr=fixdt(1,27,8)  SampleTime=-1
  Delay : Delay  DelayLength=1
  Logical Operator : Logic  AllPortsSameDT=off  OutDataTypeStr=boolean
  Logical Operator1 : Logic  Operator=NOT  AllPortsSameDT=off  OutDataTypeStr=boolean
  Multiply-Accumulate : hdlsllib/HDL Operations/Multiply-Accumulate  opMode=Streaming - using Number of Samples  initValueSetting=Dialog  initValue=0  initValueSetting2=Dialog  initValue2=0  initValueSetting3=Dialog  initValue3=0  num_samples=256  RndMeth2=Floor  RndMeth3=Floor  datatype2=Inherit: Inherit via back propagation  datatype3=fixdt(1,27,8)  validOut=on  endInandOut=on  startOut=on  countOut=on  dim=-1  DoSatur=off  parallel=off
      settings: SourceProductBaseCode=SL
  SNR : Scope  Commented=on  NumInputPorts=4
  Triggered Subsystem1 : Subsystem  TreatAsAtomicUnit=on
  SNR_check : Outport
  countOut : Outport  Port=2
  Valid_out : Outport  Port=3
  wires:
  validIn_sum/1 -> Multiply-Accumulate/3
  Constant1/1 -> Multiply-Accumulate/2
  Multiply-Accumulate/1 -> Triggered Subsystem1/1(Somme)
  " Value"/1 -> Triggered Subsystem1/2(" Valeur Max")
  Triggered Subsystem1/1(SNR check) -> Delay/1
  Multiply-Accumulate/3 -> countOut/1
  validIn_Max/1 -> Logical Operator1/1
  Logical Operator1/1 -> Logical Operator/1
  Multiply-Accumulate/2 -> Logical Operator/2
  Multiply-Accumulate/4 -> Valid_out/1
  a/1 -> Multiply-Accumulate/1
  Logical Operator/1 -> Triggered Subsystem1/Trigger
  Delay/1 -> SNR_check/1
  Triggered Subsystem1/2(Debug) -> SNR/1
  SNR_Threshold/1 -> Triggered Subsystem1/3(SNR_Threshold)

== system DOA_rearanged_2020a/Maximum Hydro 1/SampleHold ==
  Trigger : Inport
  In2 : Inport  Port=2
  Sample and Hold : dspsigops/Sample and Hold  trig=Falling edge  initCond=0  latchinput=off
  " " : Outport
  wires:
  Trigger/1 -> Sample and Hold/Trigger
  Sample and Hold/1 -> " "/1
  In2/1 -> Sample and Hold/1

== system DOA_rearanged_2020a/Maximum Hydro 1/SampleHold2 ==
  Trigger : Inport
  In2 : Inport  Port=2
  Sample and Hold : dspsigops/Sample and Hold  trig=Falling edge  initCond=0  latchinput=off
  " " : Outport
  wires:
  Trigger/1 -> Sample and Hold/Trigger
  Sample and Hold/1 -> " "/1
  In2/1 -> Sample and Hold/1

== system DOA_rearanged_2020a/Maximum Hydro 1/SampleHold3 ==
  Trigger : Inport
  In2 : Inport  Port=2
  Sample and Hold : dspsigops/Sample and Hold  trig=Falling edge  initCond=0  latchinput=off
  " " : Outport
  wires:
  Trigger/1 -> Sample and Hold/Trigger
  Sample and Hold/1 -> " "/1
  In2/1 -> Sample and Hold/1

== system DOA_rearanged_2020a/Maximum Hydro 1/SampleHold4 ==
  Trigger : Inport
  In2 : Inport  Port=2
  Sample and Hold : dspsigops/Sample and Hold  trig=Falling edge  initCond=0  latchinput=off
  " " : Outport
  wires:
  Trigger/1 -> Sample and Hold/Trigger
  Sample and Hold/1 -> " "/1
  In2/1 -> Sample and Hold/1

== system DOA_rearanged_2020a/Maximum Hydro 1/SampleHold5 ==
  Trigger : Inport
  In2 : Inport  Port=2
  Sample and Hold : dspsigops/Sample and Hold  trig=Falling edge  initCond=0  latchinput=off
  " " : Outport
  wires:
  Trigger/1 -> Sample and Hold/Trigger
  Sample and Hold/1 -> " "/1
  In2/1 -> Sample and Hold/1

== system DOA_rearanged_2020a/Maximum Hydro 1/SampleHold6 ==
  Trigger : Inport
  In2 : Inport  Port=2
  Sample and Hold : dspsigops/Sample and Hold  trig=Falling edge  initCond=0  latchinput=off
  " " : Outport
  wires:
  Trigger/1 -> Sample and Hold/Trigger
  Sample and Hold/1 -> " "/1
  In2/1 -> Sample and Hold/1

== system DOA_rearanged_2020a/Maximum Hydro 1/Subsystem ==
  Enable/Reset : Inport
  Add : Sum
  Data Type Conversion1 : DataTypeConversion  OutDataTypeStr=uint16  RndMeth=Nearest
  Delay : Delay  DelayLength=1  InitialCondition=0  UseCircularBuffer=on
  Product2 : Product
  Count : Outport  VectorParamsAs1DForOutWhenUnconnected=off
  wires:
  Enable/Reset/1 -> Add/1, Product2/1
  Add/1 -> Product2/2
  Delay/1 -> Count/1, Data Type Conversion1/1
  Product2/1 -> Delay/1
  Data Type Conversion1/1 -> Add/2

== system DOA_rearanged_2020a/Maximum Hydro 2/SampleHold ==
  Trigger : Inport
  In2 : Inport  Port=2
  Sample and Hold : dspsigops/Sample and Hold  trig=Falling edge  initCond=0  latchinput=off
  " " : Outport
  wires:
  Trigger/1 -> Sample and Hold/Trigger
  Sample and Hold/1 -> " "/1
  In2/1 -> Sample and Hold/1

== system DOA_rearanged_2020a/Maximum Hydro 2/SampleHold2 ==
  Trigger : Inport
  In2 : Inport  Port=2
  Sample and Hold : dspsigops/Sample and Hold  trig=Falling edge  initCond=0  latchinput=off
  " " : Outport
  wires:
  Trigger/1 -> Sample and Hold/Trigger
  Sample and Hold/1 -> " "/1
  In2/1 -> Sample and Hold/1

== system DOA_rearanged_2020a/Maximum Hydro 2/SampleHold3 ==
  Trigger : Inport
  In2 : Inport  Port=2
  Sample and Hold : dspsigops/Sample and Hold  trig=Falling edge  initCond=0  latchinput=off
  " " : Outport
  wires:
  Trigger/1 -> Sample and Hold/Trigger
  Sample and Hold/1 -> " "/1
  In2/1 -> Sample and Hold/1

== system DOA_rearanged_2020a/Maximum Hydro 2/SampleHold4 ==
  Trigger : Inport
  In2 : Inport  Port=2
  Sample and Hold : dspsigops/Sample and Hold  trig=Falling edge  initCond=0  latchinput=off
  " " : Outport
  wires:
  Trigger/1 -> Sample and Hold/Trigger
  Sample and Hold/1 -> " "/1
  In2/1 -> Sample and Hold/1

== system DOA_rearanged_2020a/Maximum Hydro 2/SampleHold5 ==
  Trigger : Inport
  In2 : Inport  Port=2
  Sample and Hold : dspsigops/Sample and Hold  trig=Falling edge  initCond=0  latchinput=off
  " " : Outport
  wires:
  Trigger/1 -> Sample and Hold/Trigger
  Sample and Hold/1 -> " "/1
  In2/1 -> Sample and Hold/1

== system DOA_rearanged_2020a/Maximum Hydro 2/SampleHold6 ==
  Trigger : Inport
  In2 : Inport  Port=2
  Sample and Hold : dspsigops/Sample and Hold  trig=Falling edge  initCond=0  latchinput=off
  " " : Outport
  wires:
  Trigger/1 -> Sample and Hold/Trigger
  Sample and Hold/1 -> " "/1
  In2/1 -> Sample and Hold/1

== system DOA_rearanged_2020a/Maximum Hydro 2/Subsystem ==
  Enable/Reset : Inport
  Add : Sum
  Data Type Conversion1 : DataTypeConversion  OutDataTypeStr=uint16  RndMeth=Nearest
  Delay : Delay  DelayLength=1  InitialCondition=0  UseCircularBuffer=on
  Product2 : Product
  Count : Outport  VectorParamsAs1DForOutWhenUnconnected=off
  wires:
  Enable/Reset/1 -> Add/1, Product2/1
  Add/1 -> Product2/2
  Delay/1 -> Count/1, Data Type Conversion1/1
  Product2/1 -> Delay/1
  Data Type Conversion1/1 -> Add/2

== system DOA_rearanged_2020a/Maximum Hydro 3/SampleHold ==
  Trigger : Inport
  In2 : Inport  Port=2
  Sample and Hold : dspsigops/Sample and Hold  trig=Falling edge  initCond=0  latchinput=off
  " " : Outport
  wires:
  Trigger/1 -> Sample and Hold/Trigger
  Sample and Hold/1 -> " "/1
  In2/1 -> Sample and Hold/1

== system DOA_rearanged_2020a/Maximum Hydro 3/SampleHold2 ==
  Trigger : Inport
  In2 : Inport  Port=2
  Sample and Hold : dspsigops/Sample and Hold  trig=Falling edge  initCond=0  latchinput=off
  " " : Outport
  wires:
  Trigger/1 -> Sample and Hold/Trigger
  Sample and Hold/1 -> " "/1
  In2/1 -> Sample and Hold/1

== system DOA_rearanged_2020a/Maximum Hydro 3/SampleHold3 ==
  Trigger : Inport
  In2 : Inport  Port=2
  Sample and Hold : dspsigops/Sample and Hold  trig=Falling edge  initCond=0  latchinput=off
  " " : Outport
  wires:
  Trigger/1 -> Sample and Hold/Trigger
  Sample and Hold/1 -> " "/1
  In2/1 -> Sample and Hold/1

== system DOA_rearanged_2020a/Maximum Hydro 3/SampleHold4 ==
  Trigger : Inport
  In2 : Inport  Port=2
  Sample and Hold : dspsigops/Sample and Hold  trig=Falling edge  initCond=0  latchinput=off
  " " : Outport
  wires:
  Trigger/1 -> Sample and Hold/Trigger
  Sample and Hold/1 -> " "/1
  In2/1 -> Sample and Hold/1

== system DOA_rearanged_2020a/Maximum Hydro 3/SampleHold5 ==
  Trigger : Inport
  In2 : Inport  Port=2
  Sample and Hold : dspsigops/Sample and Hold  trig=Falling edge  initCond=0  latchinput=off
  " " : Outport
  wires:
  Trigger/1 -> Sample and Hold/Trigger
  Sample and Hold/1 -> " "/1
  In2/1 -> Sample and Hold/1

== system DOA_rearanged_2020a/Maximum Hydro 3/SampleHold6 ==
  Trigger : Inport
  In2 : Inport  Port=2
  Sample and Hold : dspsigops/Sample and Hold  trig=Falling edge  initCond=0  latchinput=off
  " " : Outport
  wires:
  Trigger/1 -> Sample and Hold/Trigger
  Sample and Hold/1 -> " "/1
  In2/1 -> Sample and Hold/1

== system DOA_rearanged_2020a/Maximum Hydro 3/Subsystem ==
  Enable/Reset : Inport
  Add : Sum
  Data Type Conversion1 : DataTypeConversion  OutDataTypeStr=uint16  RndMeth=Nearest
  Delay : Delay  DelayLength=1  InitialCondition=0  UseCircularBuffer=on
  Product2 : Product
  Count : Outport  VectorParamsAs1DForOutWhenUnconnected=off
  wires:
  Enable/Reset/1 -> Add/1, Product2/1
  Add/1 -> Product2/2
  Delay/1 -> Count/1, Data Type Conversion1/1
  Product2/1 -> Delay/1
  Data Type Conversion1/1 -> Add/2

== system DOA_rearanged_2020a/Maximum Hydro Ref/SampleHold ==
  Trigger : Inport
  In2 : Inport  Port=2
  Sample and Hold : dspsigops/Sample and Hold  trig=Falling edge  initCond=0  latchinput=off
  " " : Outport
  wires:
  Trigger/1 -> Sample and Hold/Trigger
  Sample and Hold/1 -> " "/1
  In2/1 -> Sample and Hold/1

== system DOA_rearanged_2020a/Maximum Hydro Ref/SampleHold2 ==
  Trigger : Inport
  In2 : Inport  Port=2
  Sample and Hold : dspsigops/Sample and Hold  trig=Falling edge  initCond=0  latchinput=off
  " " : Outport
  wires:
  Trigger/1 -> Sample and Hold/Trigger
  Sample and Hold/1 -> " "/1
  In2/1 -> Sample and Hold/1

== system DOA_rearanged_2020a/Maximum Hydro Ref/SampleHold3 ==
  Trigger : Inport
  In2 : Inport  Port=2
  Sample and Hold : dspsigops/Sample and Hold  trig=Falling edge  initCond=0  latchinput=off
  " " : Outport
  wires:
  Trigger/1 -> Sample and Hold/Trigger
  Sample and Hold/1 -> " "/1
  In2/1 -> Sample and Hold/1

== system DOA_rearanged_2020a/Maximum Hydro Ref/SampleHold4 ==
  Trigger : Inport
  In2 : Inport  Port=2
  Sample and Hold : dspsigops/Sample and Hold  trig=Falling edge  initCond=0  latchinput=off
  " " : Outport
  wires:
  Trigger/1 -> Sample and Hold/Trigger
  Sample and Hold/1 -> " "/1
  In2/1 -> Sample and Hold/1

== system DOA_rearanged_2020a/Maximum Hydro Ref/SampleHold5 ==
  Trigger : Inport
  In2 : Inport  Port=2
  Sample and Hold : dspsigops/Sample and Hold  trig=Falling edge  initCond=0  latchinput=off
  " " : Outport
  wires:
  Trigger/1 -> Sample and Hold/Trigger
  Sample and Hold/1 -> " "/1
  In2/1 -> Sample and Hold/1

== system DOA_rearanged_2020a/Maximum Hydro Ref/SampleHold6 ==
  Trigger : Inport
  In2 : Inport  Port=2
  Sample and Hold : dspsigops/Sample and Hold  trig=Falling edge  initCond=0  latchinput=off
  " " : Outport
  wires:
  Trigger/1 -> Sample and Hold/Trigger
  Sample and Hold/1 -> " "/1
  In2/1 -> Sample and Hold/1

== system DOA_rearanged_2020a/Maximum Hydro Ref/Subsystem ==
  Enable/Reset : Inport
  Add : Sum
  Data Type Conversion1 : DataTypeConversion  OutDataTypeStr=uint16  RndMeth=Nearest
  Delay : Delay  DelayLength=1  InitialCondition=0  UseCircularBuffer=on
  Product2 : Product
  Count : Outport  VectorParamsAs1DForOutWhenUnconnected=off
  wires:
  Enable/Reset/1 -> Add/1, Product2/1
  Add/1 -> Product2/2
  Delay/1 -> Count/1, Data Type Conversion1/1
  Product2/1 -> Delay/1
  Data Type Conversion1/1 -> Add/2

== system DOA_rearanged_2020a/Signal Trigger/Fenetrage ==
  Valid_in : Inport
  Enable : Inport  Port=2
  Constant : Constant  Value=0  OutDataTypeStr=uint16  SampleTime=-1
  Direct Lookup Table (n-D) : LookupNDDirect  NumberOfTableDimensions=1  Table=Coeff_han  DiagnosticForOutOfRangeInput=Error  TableMin=[0]  TableDataTypeStr=fixdt(0,9,8)
  Subsystem : Subsystem
  Switch : Switch  Threshold=FFT_LENGTH  OutMin=[0]  OutMax=[511]  OutDataTypeStr=uint16
  coeff : Outport
  wires:
  Direct Lookup Table (n-D)/1 -> coeff/1
  Valid_in/1 -> Subsystem/1(Reset)
  Constant/1 -> Switch/1
  Enable/1 -> Subsystem/2(Enable)
  Switch/1 -> Direct Lookup Table (n-D)/1
  Subsystem/1(Count) -> Switch/3, Switch/2

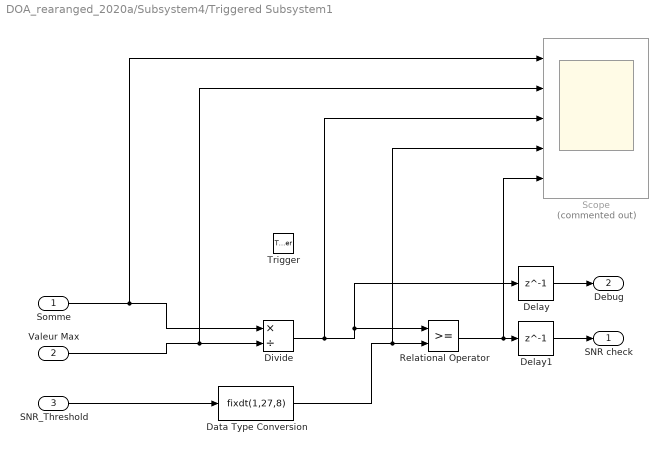
== system DOA_rearanged_2020a/Subsystem4/Triggered Subsystem1 ==
  Somme : Inport
  " Valeur Max" : Inport  Port=2
  SNR_Threshold : Inport  Port=3
  Trigger : TriggerPort  VariantControl=Variant
  Data Type Conversion : DataTypeConversion  OutDataTypeStr=fixdt(1,27,8)
  Delay : Delay  DelayLength=1
  Delay1 : Delay  DelayLength=1
  Divide : Product  Inputs=*/  RndMeth=Zero  SaturateOnIntegerOverflow=on
  Relational Operator : RelationalOperator  OutDataTypeStr=boolean  RndMeth=Simplest
  Scope : Scope  Commented=on  NumInputPorts=5
  SNR check : Outport  InitialOutput=[0]  VectorParamsAs1DForOutWhenUnconnected=off
  Debug : Outport  Port=2  InitialOutput=[0]  VectorParamsAs1DForOutWhenUnconnected=off
  wires:
  Relational Operator/1 -> Delay1/1, Scope/5
  SNR_Threshold/1 -> Data Type Conversion/1
  " Valeur Max"/1 -> Scope/2, Divide/2
  Somme/1 -> Scope/1, Divide/1
  Data Type Conversion/1 -> Scope/4, Relational Operator/2
  Divide/1 -> Scope/3, Delay/1, Relational Operator/1
  Delay/1 -> Debug/1
  Delay1/1 -> SNR check/1

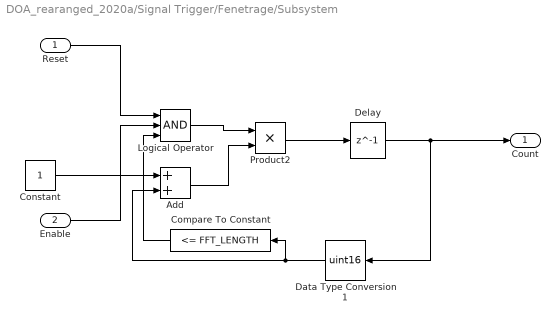
== system DOA_rearanged_2020a/Signal Trigger/Fenetrage/Subsystem ==
  Reset : Inport
  Enable : Inport  Port=2
  Add : Sum
  Compare To Constant : simulink/Logic and Bit Operations/Compare To Constant  relop=<=  const=FFT_LENGTH  OutDataTypeStr=boolean
  Constant : Constant  OutDataTypeStr=Inherit: Inherit via back propagation  SampleTime=-1
  Data Type Conversion1 : DataTypeConversion  OutDataTypeStr=uint16  RndMeth=Nearest
  Delay : Delay  DelayLength=1  InitialCondition=0  UseCircularBuffer=on
  Logical Operator : Logic  Inputs=3  AllPortsSameDT=off  OutDataTypeStr=boolean
  Product2 : Product  OutDataTypeStr=uint16
  Count : Outport  VectorParamsAs1DForOutWhenUnconnected=off
  wires:
  Delay/1 -> Count/1, Data Type Conversion1/1
  Product2/1 -> Delay/1
  Data Type Conversion1/1 -> Add/2, Compare To Constant/1
  Reset/1 -> Logical Operator/1
  Compare To Constant/1 -> Logical Operator/3
  Logical Operator/1 -> Product2/1
  Add/1 -> Product2/2
  Enable/1 -> Logical Operator/2
  Constant/1 -> Add/1
